simulink model "OneDoF_simulation"  (R2025b)
settings: Solver=ode45  StartTime=0.0  StopTime=Tend  MaxStep=1e-3  MinStep=1e-4  RelTol=1e-3
undefined symbols (not defined in the file): delta_2, rho, Ts
libraries: cstblocks x2, simulink x1
settings Model: Creator=davidecovolo  LastModifiedBy=davidecovolo
settings SolverCC: InitialStep=1e-4

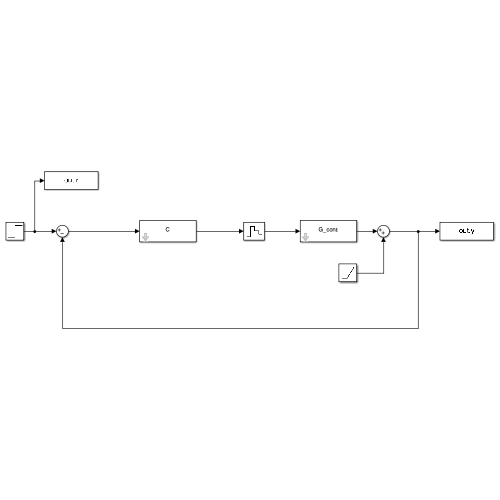
[thumbnail: Simulink's stored preview of the top-level diagram]
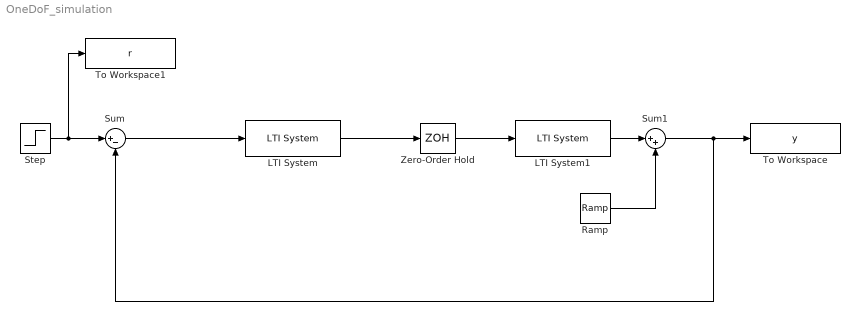
== system OneDoF_simulation ==
  LTI System : cstblocks/LTI System  sys=C  IC=[]  PadeOrder=0
  LTI System1 : cstblocks/LTI System  sys=G_cont  IC=[]  PadeOrder=0
  Ramp : simulink/Sources/Ramp  slope=delta_2  start=0  InitialOutput=0
  Step : Step  Time=0  After=rho  SampleTime=Ts
  Sum : Sum  Inputs=|+-
  Sum1 : Sum  Inputs=|++
  To Workspace : ToWorkspace  VariableName=y  SaveFormat=Timeseries  SampleTime=Ts
  To Workspace1 : ToWorkspace  VariableName=r  SaveFormat=Timeseries  SampleTime=Ts
  Zero-Order Hold : ZeroOrderHold  SampleTime=Ts
  wires:
  Sum1/1 -> Sum/2, To Workspace/1
  Sum/1 -> LTI System/1
  LTI System/1 -> Zero-Order Hold/1
  Zero-Order Hold/1 -> LTI System1/1
  LTI System1/1 -> Sum1/1
  Step/1 -> Sum/1, To Workspace1/1
  Ramp/1 -> Sum1/2
